simulink model "SIM_SAD_DEMO"  (R2025b)
settings: Solver=ode5  StartTime=0.0  StopTime=2*T  FixedStep=0.1  RelTol=1e-3
model workspace (MAT data in the model file):
  Pnull = Simulink.Parameter
  Pnull.Value = Simulink.data.Expression
  Pnull.Value.ExpressionString = "zeros(3,1)"
  Pnull.Complexity = 'real'
  Pnull.Dimensions = -1
  Pnull.DataType = 'auto'
  rho_albedo_medio = Simulink.Parameter
  rho_albedo_medio.Value = 0.3
  rho_albedo_medio.Complexity = 'real'
  rho_albedo_medio.Dimensions = [1 1]
  rho_albedo_medio.DataType = 'auto'
values from neighbouring files (symbols this model uses):
  Aree = zeros(10,1)    [SCRIPT_SAD_DEMO.m]
  base_seed = base_seed_MC + k    [SCRIPT_SAD_DEMO.m]
  c = astroConstants(5)*1e3    [SCRIPT_SAD_DEMO.m]
  draan = 1.99096871e-7    (= 1.99096871e-07)    [SCRIPT_SAD_DEMO.m]
  dwell_time = 30    [SCRIPT_SAD_DEMO.m]
  eps_att = deg2rad(0.2)    [SCRIPT_SAD_DEMO.m]
  eps_E = deg2rad(astroConstants(63))    [SCRIPT_SAD_DEMO.m]
  eps_h_r = 0.001    [SCRIPT_SAD_DEMO.m]
  eps_w = deg2rad(0.1)    [SCRIPT_SAD_DEMO.m]
  err_max = deg2rad(15)    [SCRIPT_SAD_DEMO.m]
  F_e = 1358    [SCRIPT_SAD_DEMO.m]
  h_r_max = 0.05    [SCRIPT_SAD_DEMO.m]
  h_r_safe = 0.001    [SCRIPT_SAD_DEMO.m]
  j_B = [0.01; 0.05; 0.01]    [SCRIPT_SAD_DEMO.m]
  J_depl = J_nom    [SCRIPT_SAD_DEMO.m]
  JD0 = juliandate(startTime)    [SCRIPT_SAD_DEMO.m]
  k_b = 200000    [SCRIPT_SAD_DEMO.m]
  Kd = K(:, 1:3)    [SCRIPT_SAD_DEMO.m]
  kep = [a,e,incl,raan,w,theta]    [SCRIPT_SAD_DEMO.m]
  Kp = K(:, 4:6)    [SCRIPT_SAD_DEMO.m]
  mu = astroConstants(13)    [SCRIPT_SAD_DEMO.m]
  n = sqrt( (mu/ (a)^3))    [SCRIPT_SAD_DEMO.m]
  n_sun = 2*pi/T_sun    (= 1.99238499086e-07)    [SCRIPT_SAD_DEMO.m]
  Nmat = [ ... (first row only)    [SCRIPT_SAD_DEMO.m]
  r_sun = 1*AU    [SCRIPT_SAD_DEMO.m]
  Re = astroConstants(23)    [SCRIPT_SAD_DEMO.m]
  rf = [ ... (first row only)    [SCRIPT_SAD_DEMO.m]
  rhod = 0.1*ones(10,1)    [SCRIPT_SAD_DEMO.m]
  rhos = zeros(10,1)    [SCRIPT_SAD_DEMO.m]
  SRP = SRP_nom    [SCRIPT_SAD_DEMO.m]
  theta = 0    [SCRIPT_SAD_DEMO.m]
  w0 = w0_nom    [SCRIPT_SAD_DEMO.m]
  w_enter = Control.w_tumbling    [SCRIPT_SAD_DEMO.m]
  w_enter_2 = Control.w_pointing    [SCRIPT_SAD_DEMO.m]
  w_exit = deg2rad(4)    [SCRIPT_SAD_DEMO.m]
  w_exit_2 = deg2rad(1.5)    [SCRIPT_SAD_DEMO.m]
undefined symbols (not defined in the file or in its folder): DiscIntNeverNeededParam, Filter, Gyro, Magmeter, MTQ, q, RW, Sun_sensor
libraries: matrix_library x41, LIBRARY_SAD x40, simulink x1, cstblocks x1
(part 1 of 4)
settings Model: Creator=fabio  LastModifiedBy=delil

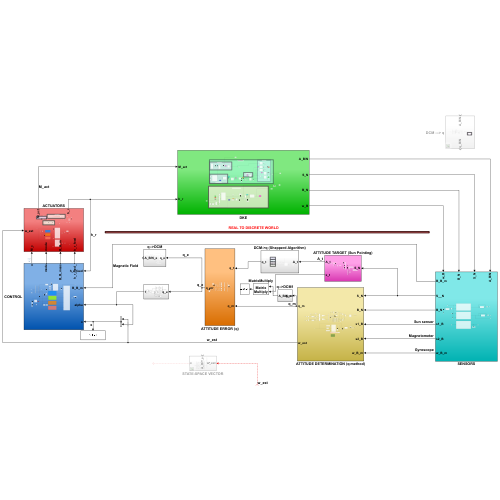
[thumbnail: Simulink's stored preview of the top-level diagram]
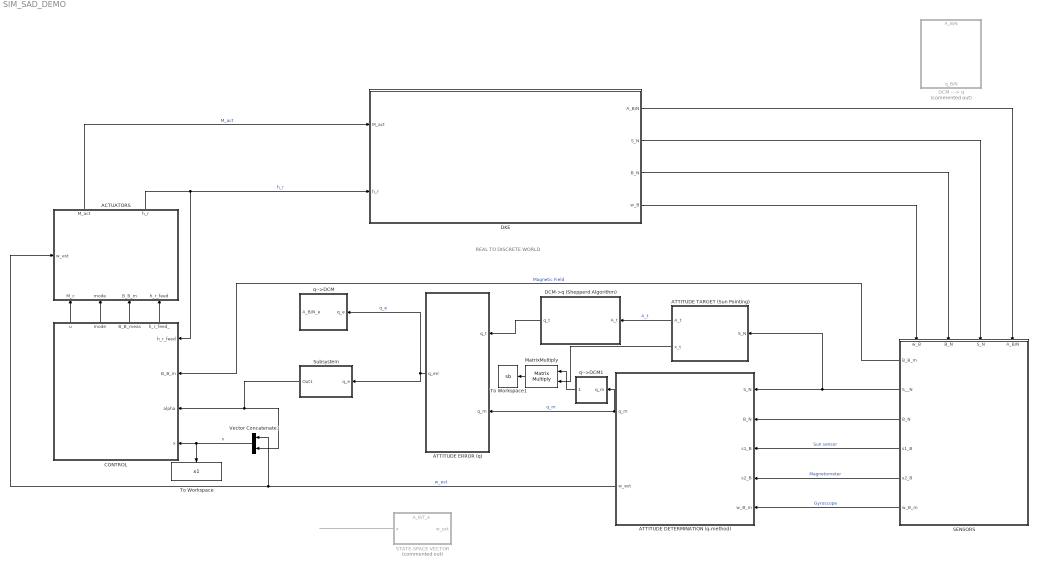
== system SIM_SAD_DEMO ==
  note: REAL TO DISCRETE WORLD
  ACTUATORS : Subsystem
      settings: PortSchema="{\"entries\":[{\"content\":{\"sides\":[{\"content\":{\"connectorIds\":[\"In1\",\"In2\",\"In3\",\"In4\"]},\"type\":\"ConnectorPlacement.EquallySpacedRectSide\",\"uuid\":\"6f22ed06-999b-49a4-bbcf-c00740f0bb3e\"},{\"content\":{\"connectorIds\":[\"Out1\",\"Out2\"],\"side\":\"RIGHT\"},\"type\":\"ConnectorPlacement.EquallySpacedRectSide\",\"uuid\":\"a2723920-c354-4b44-95a5-a047723a6fce\"},{\"content\":{\"connectorIds\":[\"In5\"],\"side\":\"TOP\"},\"type\":\"ConnectorPlacement.EquallySpacedRectSide\",\"uuid\":\"3a79ee58-4fdd-4e66-816d-19ecec84d660\"},{\"content\":{\"side\":\"BOTTOM\"},\"type\":\"ConnectorPlacement.EquallySpacedRectSide\",\"uuid\":\"88529345-5c62-4e9f-9741-99c35e09ad49\"}]},\"type\":\"ConnectorPlacement.EquallySpacedConnector\",\"uuid\":\"ec6e585e-60d6-43a1-884b-cd7dbc18dea8\"}],\"packageUris\":[\"http://schema.mathworks.com/mf0/Connector/R2020b\"],\"version\":\"1.0\"}"
  ATTITUDE DETERMINATION (q-method) : Subsystem
  ATTITUDE ERROR (q) : Subsystem
  ATTITUDE TARGET (Sun Pointing) : Subsystem
  CONTROL : Subsystem
      settings: PortSchema="{\"entries\":[{\"content\":{\"sides\":[{\"content\":{},\"type\":\"ConnectorPlacement.EquallySpacedRectSide\",\"uuid\":\"883b2e58-b302-40a6-9310-8bc36577f20a\"},{\"content\":{\"connectorIds\":[\"Out1\",\"Out2\",\"Out3\",\"Out4\"],\"side\":\"RIGHT\"},\"type\":\"ConnectorPlacement.EquallySpacedRectSide\",\"uuid\":\"3f5ac81e-dbcc-48df-b297-a852c6b84cd5\"},{\"content\":{\"side\":\"TOP\"},\"type\":\"ConnectorPlacement.EquallySpacedRectSide\",\"uuid\":\"b9661aa9-e9e6-4933-8b5a-68fb8ed8b613\"},{\"content\":{\"connectorIds\":[\"In1\",\"In2\",\"In3\",\"In4\"],\"side\":\"BOTTOM\"},\"type\":\"ConnectorPlacement.EquallySpacedRectSide\",\"uuid\":\"f58abdc6-33e7-496f-818d-03ad59e960e0\"}]},\"type\":\"ConnectorPlacement.EquallySpacedConnector\",\"uuid\":\"d8cd4486-f7c8-49c6-99e5-77f1928d07fe\"}],\"packageUris\":[\"http://schema.mathworks.com/mf0/Connector/R2020b\"],\"version\":\"1.0\"}"
  DCM ---> q : Subsystem  Commented=on
  DCM->q (Shepperd Algorithm) : Subsystem
  DKE : Subsystem
  MatrixMultiply : Product  Multiplication=Matrix(*)
  SENSORS : Subsystem
      settings: PortSchema="{\"entries\":[{\"content\":{\"sides\":[{\"content\":{\"connectorIds\":[\"In1\",\"In2\",\"In3\",\"In4\"]},\"type\":\"ConnectorPlacement.EquallySpacedRectSide\",\"uuid\":\"40962b30-3bcb-49e0-bc68-6aa3a31cfc97\"},{\"content\":{\"side\":\"RIGHT\"},\"type\":\"ConnectorPlacement.EquallySpacedRectSide\",\"uuid\":\"a8221d80-3d13-495d-884e-34f2ccc75f25\"},{\"content\":{\"connectorIds\":[\"Out1\",\"Out2\",\"Out3\",\"Out4\",\"Out5\",\"Out6\"],\"side\":\"TOP\"},\"type\":\"ConnectorPlacement.EquallySpacedRectSide\",\"uuid\":\"62b0f620-b15f-4d6a-bcfa-939a48d36217\"}]},\"type\":\"ConnectorPlacement.EquallySpacedConnector\",\"uuid\":\"bc93d320-282b-4258-8528-17688a47c52b\"}],\"packageUris\":[\"http://schema.mathworks.com/mf0/Connector/R2020b\"],\"version\":\"1.0\"}"
  STATE-SPACE VECTOR : Subsystem  Commented=on
      settings: PortSchema="{\"entries\":[{\"content\":{\"sides\":[{\"content\":{\"connectorIds\":[\"In1\"]},\"type\":\"ConnectorPlacement.EquallySpacedRectSide\",\"uuid\":\"179348e5-c488-47fb-b567-6c698cd263cb\"},{\"content\":{\"connectorIds\":[\"Out1\"],\"side\":\"RIGHT\"},\"type\":\"ConnectorPlacement.EquallySpacedRectSide\",\"uuid\":\"b2471475-7911-4c4c-b1de-354e85644b05\"},{\"content\":{\"connectorIds\":[\"In2\"],\"side\":\"TOP\"},\"type\":\"ConnectorPlacement.EquallySpacedRectSide\",\"uuid\":\"d61f0b2a-82cf-4d0f-843a-7dc5d306adfe\"},{\"content\":{\"side\":\"BOTTOM\"},\"type\":\"ConnectorPlacement.EquallySpacedRectSide\",\"uuid\":\"cf78bb57-5448-49c7-a009-bc1da3dda3c1\"}]},\"type\":\"ConnectorPlacement.EquallySpacedConnector\",\"uuid\":\"246de782-537f-47b1-b071-25d14f8cca05\"}],\"packageUris\":[\"http://schema.mathworks.com/mf0/Connector/R2020b\"],\"version\":\"1.0\"}"
  Subsystem : Subsystem
  To Workspace : ToWorkspace  VariableName=x1  SampleTime=-1
  To Workspace1 : ToWorkspace  VariableName=sb  SampleTime=-1
  Vector Concatenate1 : Concatenate
  q-->DCM : Subsystem
  q-->DCM1 : Subsystem
  wires:
  MatrixMultiply/1 -> To Workspace1/1
  SENSORS/1(B_B_m) -> CONTROL/3(B_B_m)  "Magnetic Field"
  Vector Concatenate1/1 -> To Workspace/1, CONTROL/1(x)  "x"
  DKE/1(A_B/N) -> SENSORS/4(A_B/N)
  DKE/2(S_N) -> SENSORS/3(S_N)
  SENSORS/3(B_N) -> ATTITUDE DETERMINATION (q-method)/2(B_N)
  CONTROL/2(mode) -> ACTUATORS/2(mode)
  ATTITUDE TARGET (Sun Pointing)/1(A_t) -> DCM->q (Shepperd Algorithm)/1(A_t)  "A_t"
  ATTITUDE DETERMINATION (q-method)/1(q_m) -> ATTITUDE ERROR (q)/2(q_m), q-->DCM1/1(q_m)  "q_m"
  CONTROL/4(h_r_feed_) -> ACTUATORS/4(h_r_feed)
  SENSORS/5(s2_B) -> ATTITUDE DETERMINATION (q-method)/4(s2_B)  "Magnetometer"
  DKE/4(w_B) -> SENSORS/1(w_B)
  SENSORS/2(S__N) -> ATTITUDE TARGET (Sun Pointing)/1(S_N), ATTITUDE DETERMINATION (q-method)/1(S_N)
  ATTITUDE ERROR (q)/1(q_err) -> q-->DCM/1(q_e), Subsystem/1(q_e)  "q_e"
  DCM->q (Shepperd Algorithm)/1(q_t) -> ATTITUDE ERROR (q)/1(q_t)
  Subsystem/1(Out1) -> Vector Concatenate1/2, CONTROL/2(alpha)
  CONTROL/1(u) -> ACTUATORS/1(M_c)
  ACTUATORS/1(M_act) -> DKE/1(M_act)  "M_act"
  CONTROL/3(B_B_meas) -> ACTUATORS/3(B_B_m)
  SENSORS/6(w_B_m) -> ATTITUDE DETERMINATION (q-method)/5(w_B_m)  "Gyroscope"
  ? -> STATE-SPACE VECTOR/1(w_est)  "w_est"
  ATTITUDE TARGET (Sun Pointing)/2(x_t) -> MatrixMultiply/2
  DKE/3(B_N) -> SENSORS/2("B_N ")
  ACTUATORS/2(h_r) -> DKE/2(h_r), CONTROL/4(h_r_feed)  "h_r"
  ATTITUDE DETERMINATION (q-method)/2(w_est) -> ACTUATORS/5(w_est), Vector Concatenate1/1  "w_est"
  STATE-SPACE VECTOR/1(x) -> ?
  SENSORS/4(s1_B) -> ATTITUDE DETERMINATION (q-method)/3(s1_B)  "Sun sensor"
  q-->DCM1/1(A_B/N_m) -> MatrixMultiply/1

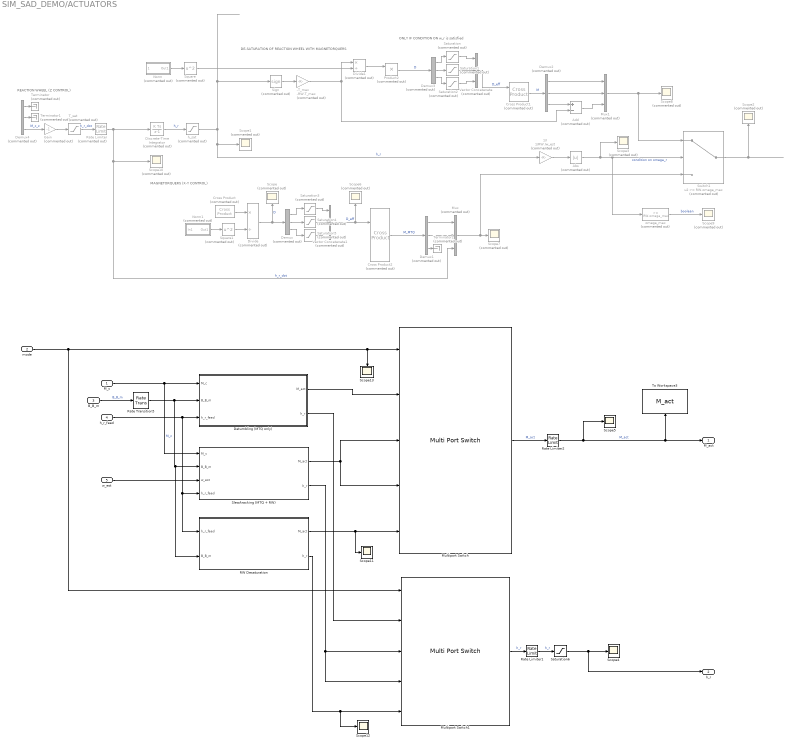
== system SIM_SAD_DEMO/ACTUATORS ==
  note: ONLY IF CONDITION ON w_r is satisfied
  note: DE-SATURATION OF REACTION WHEEL WITH MAGNETORQUERS
  note: REACTION WHEEL (Z CONTROL)
  note: MAGNETORQUERS (X-Y CONTROL)
  M_c : Inport
  mode : Inport  Port=2
  B_B_m : Inport  Port=3
  h_r_feed : Inport  Port=4
  w_est : Inport  Port=5
  -T_max : Gain  Commented=on  Gain=-RW.T_max
  1/I : Gain  Commented=on  Gain=1/RW.Iw_est
  Abs : Abs  Commented=on  SaturateOnIntegerOverflow=off
  Add : Sum  Commented=on  Inputs=+-
  Cross Product : matrix_library/Cross Product  Commented=on
  Cross Product1 : matrix_library/Cross Product  Commented=on
  Cross Product2 : matrix_library/Cross Product  Commented=on
  Demux{,1..4} (5 alike) : Demux  Commented=on  Outputs=3
  Detumbling (MTQ only) : Subsystem
  Discrete-Time Integrator : DiscreteIntegrator  Commented=on  SampleTime=-1  ICPrevOutput=DiscIntNeverNeededParam  ICPrevScaledInput=DiscIntNeverNeededParam
  Divide : Product  Commented=on  Inputs=*/
  Divide1 : Product  Commented=on  Inputs=*/
  Gain : Gain  Commented=on  Gain=-1
  Multiport Switch : MultiPortSwitch  Inputs=4  DiagnosticForDefault=None  SaturateOnIntegerOverflow=off  InputSameDT=off
  Multiport Switch1 : MultiPortSwitch  Inputs=4  DiagnosticForDefault=None  SaturateOnIntegerOverflow=off  InputSameDT=off
  Mux : Mux  Commented=on  Inputs=3
  Mux1 : Mux  Commented=on  Inputs=3
  Norm : Subsystem  Commented=on
  Norm1 : Subsystem  Commented=on
  Product2 : Product  Commented=on
  RW Desaturation : Subsystem
  Rate Limiter : RateLimiter  Commented=on  RisingSlewLimit=200  FallingSlewLimit=-200  SampleTimeMode=inherited
  Rate Limiter1 : RateLimiter  SampleTimeMode=inherited
  Rate Limiter2 : RateLimiter  SampleTimeMode=inherited
  Rate Transition5 : RateTransition  OutPortSampleTime=max([Sun_sensor.Ts,Magmeter.Ts,Gyro.Ts])
  Saturation{,1,3..4} (4 alike) : Saturate  Commented=on  UpperLimit=MTQ.D_max_XY  LowerLimit=-MTQ.D_max_XY
  Saturation2 : Saturate  Commented=on  UpperLimit=MTQ.D_max_Z  LowerLimit=-MTQ.D_max_Z
  Saturation5 : Saturate  Commented=on  UpperLimit=MTQ.D_max_Z  LowerLimit=-MTQ.D_max_Z
  Saturation6 : Saturate  UpperLimit=RW.h_max  LowerLimit=-RW.h_max
  Scope{,1..3,6..10} (9 alike) : Scope  Commented=on
      Scope settings: ActiveDisplayYMinimum=-14.411553950631344  ActiveDisplayYMaximum=16.201380468990443  DataLoggingVariableName=ScopeData98
      Scope1 settings: ActiveDisplayYMinimum=-0.0062499999999999986  ActiveDisplayYMaximum=0.05625  DataLoggingVariableName=ScopeData104
      Scope10 settings: ActiveDisplayYMinimum=-0.0099459564386370769  ActiveDisplayYMaximum=0.0095136079477336766  DataLoggingVariableName=ScopeData110
      Scope2 settings: ActiveDisplayYMinimum=-9.87718527241468E-5  ActiveDisplayYMaximum=8.9550339314577583E-5  DataLoggingVariableName=ScopeData102
      Scope3 settings: ActiveDisplayYMinimum=-65.022890693082175  ActiveDisplayYMaximum=585.20601623773973  DataLoggingVariableName=ScopeData60
      Scope6 settings: ActiveDisplayYMinimum=-0.625  ActiveDisplayYMaximum=0.625  DataLoggingVariableName=ScopeData101
      Scope7 settings: ActiveDisplayYMinimum=-1  ActiveDisplayYMaximum=1  DataLoggingVariableName=ScopeData100
      Scope8 settings: ActiveDisplayYMinimum=-0.001101814270019531  ActiveDisplayYMaximum=0.00911127471923828  DataLoggingVariableName=ScopeData103
      Scope9 settings: ActiveDisplayYMinimum=-0.12499999999999997  ActiveDisplayYMaximum=1.125  DataLoggingVariableName=ScopeData107
  Scope{4..5,11..13} (5 alike) : Scope
      Scope11 settings: ActiveDisplayYMinimum=-1  ActiveDisplayYMaximum=1  DataLoggingVariableName=ScopeData119
      Scope12 settings: ActiveDisplayYMinimum=-1  ActiveDisplayYMaximum=1  DataLoggingVariableName=ScopeData121
      Scope13 settings: ActiveDisplayYMinimum=-0.49999999999999989  ActiveDisplayYMaximum=4.5  DataLoggingVariableName=ScopeData125
      Scope4 settings: ActiveDisplayYMinimum=-0.0625  ActiveDisplayYMaximum=0.0625  DataLoggingVariableName=ScopeData114
      Scope5 settings: ActiveDisplayYMinimum=-1.2499999497669214  ActiveDisplayYMaximum=1.2499999579450596  DataLoggingVariableName=ScopeData115
  Sign : Signum  Commented=on
  Slew/tracking (MTQ + RW) : Subsystem
  Square : Math  Commented=on  Operator=square
  Square1 : Math  Commented=on  Operator=square
  Switch1 : Switch  Commented=on  Threshold=RW.omega_max  SaturateOnIntegerOverflow=off  InputSameDT=off
  T_sat : Saturate  Commented=on  UpperLimit=RW.T_max  LowerLimit=-RW.T_max
  Terminator : Terminator  Commented=on
  Terminator1 : Terminator  Commented=on
  Terminator2 : Terminator  Commented=on
  To Workspace3 : ToWorkspace  VariableName=M_act  SampleTime=-1
  Vector Concatenate : Concatenate  Commented=on  NumInputs=3
  Vector Concatenate1 : Concatenate  Commented=on  NumInputs=3
  h_sat : Saturate  Commented=on  UpperLimit=RW.h_max  LowerLimit=-RW.h_max
  omega_max : simulink/Logic and Bit Operations/Compare To Constant  Commented=on  relop=>=  const=RW.omega_max  OutDataTypeStr=boolean
  M_act : Outport
  h_r : Outport  Port=2
  wires:
  Discrete-Time Integrator/1 -> h_sat/1  "h_r"
  Demux3/1 -> Saturation/1
  Demux3/3 -> Saturation2/1
  Product2/1 -> Demux3/1  "D"
  Divide1/1 -> Product2/1
  -T_max/1 -> Add/2, Divide1/1
  Mux1/1 -> Scope8/1, Switch1/1
  Norm/1(Out1) -> Square/1
  Saturation2/1 -> Vector Concatenate/3
  Saturation/1 -> Vector Concatenate/1
  Cross Product1/1 -> Demux2/1  "M"
  Vector Concatenate/1 -> Cross Product1/1  "D_eff"
  Demux3/2 -> Saturation1/1
  Add/1 -> Mux1/3
  Sign/1 -> -T_max/1
  T_sat/1 -> Rate Limiter/1  "h_r_dot"
  ? -> Norm1/1(In1), Cross Product/1, Cross Product2/2, Cross Product1/2, Product2/2, Norm/1(B_B_m)  "B_B_m"
  Demux4/3 -> Gain/1  "M_c_z"
  Demux2/3 -> Add/1
  Demux2/2 -> Mux1/2
  Demux2/1 -> Mux1/1
  1/I/1 -> Abs/1
  Abs/1 -> omega_max/1, Switch1/2, Scope3/1  "condition on omega_r"
  Saturation1/1 -> Vector Concatenate/2
  Cross Product/1 -> Divide/1
  Demux/1 -> Saturation3/1
  Vector Concatenate1/1 -> Cross Product2/1, Scope6/1  "D_eff"
  Saturation4/1 -> Vector Concatenate1/2
  Square1/1 -> Divide/2
  Norm1/1(Out1) -> Square1/1
  ? -> Demux4/1, Cross Product/2  "M_c"
  Divide/1 -> Scope/1, Demux/1  "D"
  Demux/2 -> Saturation4/1
  Saturation3/1 -> Vector Concatenate1/1
  Demux/3 -> Saturation5/1
  omega_max/1 -> Scope9/1  "boolean"
  Square/1 -> Divide1/2
  Saturation5/1 -> Vector Concatenate1/3
  Cross Product2/1 -> Demux1/1  "M_MTQ"
  Demux1/1 -> Mux/1
  Demux1/2 -> Mux/2
  Mux/1 -> Scope7/1, Switch1/3
  Demux4/1 -> Terminator/1
  Demux4/2 -> Terminator1/1
  Demux1/3 -> Terminator2/1
  Switch1/1 -> Scope2/1
  h_sat/1 -> Sign/1, Scope1/1, 1/I/1  "h_r"
  Rate Limiter/1 -> Discrete-Time Integrator/1, Mux/3, Scope10/1  "h_r_dot"
  Gain/1 -> T_sat/1
  M_c/1 -> Slew/tracking (MTQ + RW)/1(M_c), Detumbling (MTQ only)/1(M_c)  "M_c"
  B_B_m/1 -> Rate Transition5/1  "B_B_m"
  h_r_feed/1 -> RW Desaturation/1(h_r_feed), Slew/tracking (MTQ + RW)/4(h_r_feed), Detumbling (MTQ only)/3(h_r_feed)
  Detumbling (MTQ only)/1(M_act) -> Multiport Switch/2
  Detumbling (MTQ only)/2(h_r) -> Multiport Switch1/2
  Multiport Switch/1 -> Rate Limiter2/1  "M_act"
  Multiport Switch1/1 -> Rate Limiter1/1  "h_r"
  w_est/1 -> Slew/tracking (MTQ + RW)/3(w_est)
  Slew/tracking (MTQ + RW)/1(M_act) -> Multiport Switch/4, Multiport Switch/3
  Slew/tracking (MTQ + RW)/2(h_r) -> Multiport Switch1/3, Multiport Switch1/4
  Rate Limiter1/1 -> Saturation6/1  "h_r"
  Rate Limiter2/1 -> Scope5/1, M_act/1, To Workspace3/1  "M_act"
  Saturation6/1 -> h_r/1, Scope4/1
  mode/1 -> Multiport Switch1/1, Multiport Switch/1, Scope13/1
  RW Desaturation/1(M_act) -> Multiport Switch/5, Scope11/1
  RW Desaturation/2(h_r) -> Multiport Switch1/5, Scope12/1
  Rate Transition5/1 -> RW Desaturation/2(B_B_m), Slew/tracking (MTQ + RW)/2(B_B_m), Detumbling (MTQ only)/2(B_B_m)

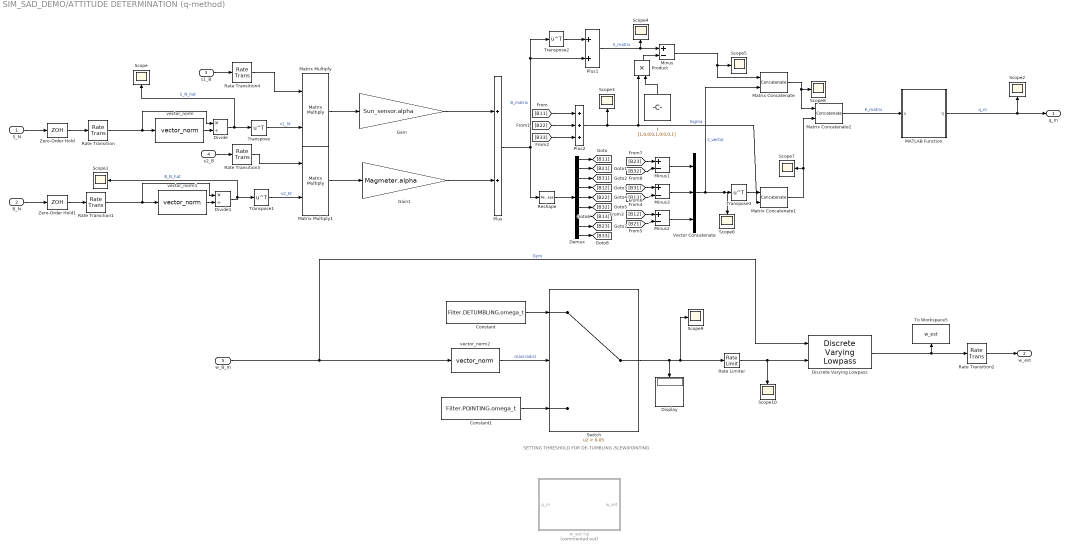
== system SIM_SAD_DEMO/ATTITUDE DETERMINATION (q-method) ==
  note: SETTING THRESHOLD FOR DE-TUMBLING /SLEW/POINTING
  S_N : Inport
  B_N : Inport  Port=2
  s1_B : Inport  Port=3
  s2_B : Inport  Port=4
  w_B_m : Inport  Port=5
  Constant : Constant  Value=Filter.DETUMBLING.omega_t
  Constant1 : Constant  Value=Filter.POINTING.omega_t
  Demux : Demux  Outputs=9
  Discrete Varying Lowpass : cstblocks/Linear Parameter Varying/Discrete Varying Lowpass  N=1  w0=0  Ts=Gyro.Ts
  Display : Display
  Divide : Product  Inputs=*/
  Divide1 : Product  Inputs=*/
  Gain : Gain  Gain=Sun_sensor.alpha
  Gain1 : Gain  Gain=Magmeter.alpha
  I : Constant  Value=[1,0,0;0,1,0;0,0,1]
  MATLAB Function : MATLAB Function  TreatAsAtomicUnit=on  SystemSampleTime=q.Ts
  Matrix Concatenate : Concatenate  Mode=Multidimensional array  ConcatenateDimension=2
  Matrix Concatenate1 : Concatenate  Mode=Multidimensional array  ConcatenateDimension=2
  Matrix Concatenate2 : Concatenate  Mode=Multidimensional array
  Matrix Multiply : Product  Multiplication=Matrix(*)
  Matrix Multiply1 : Product  Multiplication=Matrix(*)
  Minus{,1..3} (4 alike) : Sum  Inputs=+-
  Plus : Sum
  Plus1 : Sum
  Plus2 : Sum  Inputs=+++
  Product : Product
  Rate Limiter : RateLimiter  RisingSlewLimit=5  FallingSlewLimit=-5  SampleTimeMode=inherited  InitialCondition=Filter.DETUMBLING.omega_t
  Rate Transition{,1..4} (5 alike) : RateTransition  OutPortSampleTime=max([Sun_sensor.Ts,Magmeter.Ts,Gyro.Ts])
  Reshape : Reshape  OutputDimensionality=Customize  OutputDimensions=[9,1]
  Scope{,1..10} (11 alike) : Scope
      Scope settings: ActiveDisplayYMinimum=-0.12499999999999997  ActiveDisplayYMaximum=1.125  DataLoggingVariableName=ScopeData61
      Scope1 settings: ActiveDisplayYMinimum=-0.60786913937993192  ActiveDisplayYMaximum=1.0990417923572595  DataLoggingVariableName=ScopeData62
      Scope10 settings: ActiveDisplayYMinimum=0.40419161676646631  ActiveDisplayYMaximum=9.3562874251497  DataLoggingVariableName=ScopeData58
      Scope2 settings: ActiveDisplayYMinimum=-0.9533532616313245  ActiveDisplayYMaximum=1.1062124291352333  DataLoggingVariableName=ScopeData74
      Scope3 settings: ActiveDisplayYMinimum=-1  ActiveDisplayYMaximum=1  DataLoggingVariableName=ScopeData75
      Scope4 settings: DataLoggingVariableName=ScopeData76
      Scope5 settings: ActiveDisplayYMinimum=-1  ActiveDisplayYMaximum=1  DataLoggingVariableName=ScopeData77
      Scope6 settings: DataLoggingVariableName=ScopeData78
      Scope7 settings: ActiveDisplayYMinimum=-1  ActiveDisplayYMaximum=1  DataLoggingVariableName=ScopeData79
      Scope8 settings: ActiveDisplayYMinimum=-1.2343387282561236  ActiveDisplayYMaximum=1.1812725103052406  DataLoggingVariableName=ScopeData80
      Scope9 settings: ActiveDisplayYMinimum=-0.12499999999999978  ActiveDisplayYMaximum=11.125  DataLoggingVariableName=ScopeData85
  Switch : Switch  Criteria=u2 > Threshold  Threshold=0.05  SaturateOnIntegerOverflow=off  InputSameDT=off
  To Workspace5 : ToWorkspace  VariableName=w_est  SampleTime=-1
  Transpose{,1..3} (4 alike) : Math  Operator=transpose
  Vector Concatenate : Concatenate  NumInputs=3
  Zero-Order Hold : ZeroOrderHold  SampleTime=max([Sun_sensor.Ts,Magmeter.Ts,Gyro.Ts])
  Zero-Order Hold1 : ZeroOrderHold  SampleTime=max([Sun_sensor.Ts,Magmeter.Ts,Gyro.Ts])
  vector_norm : LIBRARY_SAD/vector_norm  SystemSampleTime=-1  VariantActivationTime=update diagram  EmptyChoice=off  PassThrough=off  PassThroughVariantControl=(default)  EmptyChoiceVariantControl=(default)  AllowFlexibleInterface=on  Latency=0  AutoFrameSizeCalculation=off
  vector_norm1 : LIBRARY_SAD/vector_norm  SystemSampleTime=-1  VariantActivationTime=update diagram  EmptyChoice=off  PassThrough=off  PassThroughVariantControl=(default)  EmptyChoiceVariantControl=(default)  AllowFlexibleInterface=on  Latency=0  AutoFrameSizeCalculation=off
  vector_norm2 : LIBRARY_SAD/vector_norm  SystemSampleTime=-1  VariantActivationTime=update diagram  EmptyChoice=off  PassThrough=off  PassThroughVariantControl=(default)  EmptyChoiceVariantControl=(default)  AllowFlexibleInterface=on  Latency=0  AutoFrameSizeCalculation=off
  w_est (q) : Subsystem  Commented=on
  q_m : Outport
  w_est : Outport  Port=2
  wires:
  vector_norm/1 -> Divide/2
  Demux/6 -> [B32]
  Divide/1 -> Scope/1, Transpose/1  "S_N_hat"
  Gain/1 -> Plus/1
  [B32] -> Minus1/2
  Gain1/1 -> Plus/2
  S_N/1 -> Zero-Order Hold/1
  Plus2/1 -> Scope3/1, Product/1, Matrix Concatenate1/2  "Sigma"
  B_N/1 -> Zero-Order Hold1/1
  Demux/4 -> [B12]
  Plus/1 -> Reshape/1, Transpose2/1, Plus1/2  "B_matrix"
  Divide1/1 -> Scope1/1, Transpose1/1  "B_N_hat"
  [B12] -> Minus2/1
  Demux/3 -> [B31]
  Demux/8 -> [B23]
  Vector Concatenate/1 -> Matrix Concatenate/2, Transpose3/1, Scope6/1  "z_vector"
  Minus1/1 -> Vector Concatenate/1
  Minus2/1 -> Vector Concatenate/3
  Transpose2/1 -> Plus1/1
  [B11] -> Plus2/1
  Transpose/1 -> Matrix Multiply/2  "v1_N'"
  Minus/1 -> Scope5/1, Matrix Concatenate/1
  Matrix Concatenate1/1 -> Scope7/1, Matrix Concatenate2/2
  Demux/1 -> [B11]
  [B22] -> Plus2/2
  Matrix Multiply1/1 -> Gain1/1
  Demux/2 -> [B21]
  [B23] -> Minus1/1
  Demux/5 -> [B22]
  Matrix Multiply/1 -> Gain/1
  Demux/9 -> [B33]
  Reshape/1 -> Demux/1
  Demux/7 -> [B13]
  vector_norm1/1 -> Divide1/2
  [B33] -> Plus2/3
  Matrix Concatenate/1 -> Matrix Concatenate2/1, Scope8/1
  Transpose1/1 -> Matrix Multiply1/2  "v2_N'"
  Transpose3/1 -> Matrix Concatenate1/1
  Minus3/1 -> Vector Concatenate/2
  [B31] -> Minus3/1
  Plus1/1 -> Minus/1, Scope4/1  "S_matrix"
  [B13] -> Minus3/2
  [B21] -> Minus2/2
  Product/1 -> Minus/2
  I/1 -> Product/2
  s1_B/1 -> Rate Transition4/1
  s2_B/1 -> Rate Transition3/1
  MATLAB Function/1(q) -> q_m/1, Scope2/1  "q_m"
  Switch/1 -> Rate Limiter/1, Scope9/1, Display/1
  Matrix Concatenate2/1 -> MATLAB Function/1(u)  "K_matrix"
  vector_norm2/1 -> Switch/2  "max(rad/s)"
  w_B_m/1 -> vector_norm2/1, Discrete Varying Lowpass/1  "Gyro"
  Discrete Varying Lowpass/1 -> To Workspace5/1, Rate Transition2/1
  Constant/1 -> Switch/1
  Constant1/1 -> Switch/3
  Rate Limiter/1 -> Scope10/1, Discrete Varying Lowpass/2
  Rate Transition/1 -> Divide/1, vector_norm/1
  Rate Transition1/1 -> Divide1/1, vector_norm1/1
  Rate Transition3/1 -> Matrix Multiply1/1
  Rate Transition4/1 -> Matrix Multiply/1
  Zero-Order Hold/1 -> Rate Transition/1
  Zero-Order Hold1/1 -> Rate Transition1/1
  Rate Transition2/1 -> w_est/1

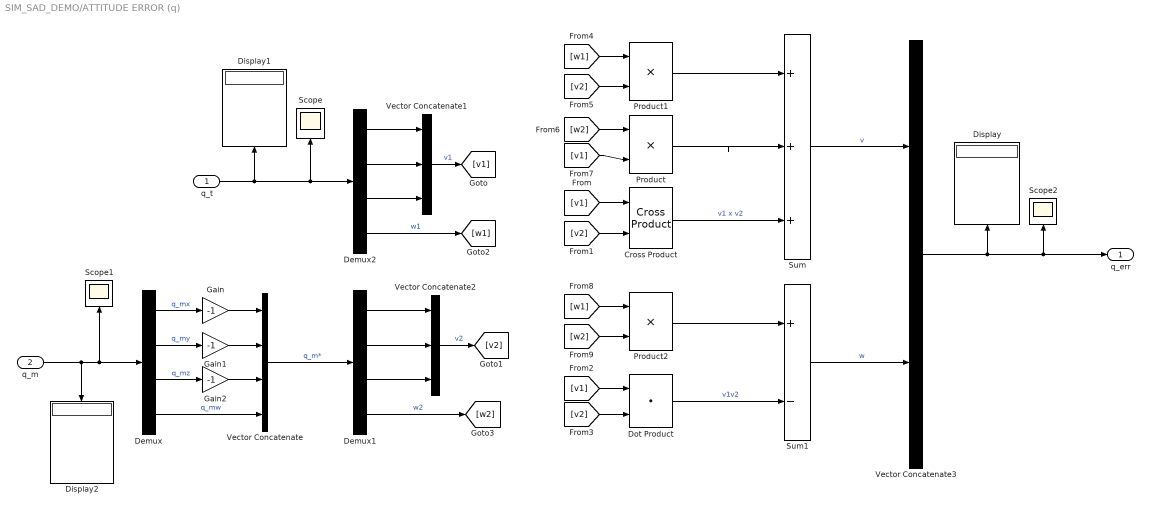
== system SIM_SAD_DEMO/ATTITUDE ERROR (q) ==
  q_t : Inport
  q_m : Inport  Port=2
  Cross Product : matrix_library/Cross Product
  Demux : Demux
  Demux1 : Demux
  Demux2 : Demux
  Display : Display
  Display1 : Display
  Display2 : Display
  Dot Product : DotProduct  OutDataTypeStr=Inherit: Inherit via internal rule
  Gain : Gain  Gain=-1
  Gain1 : Gain  Gain=-1
  Gain2 : Gain  Gain=-1
  Product : Product
  Product1 : Product
  Product2 : Product
  Scope : Scope
      settings: ActiveDisplayYMinimum=-0.12923710595911297  ActiveDisplayYMaximum=1.1085905151201327  DataLoggingVariableName=ScopeData63
  Scope1 : Scope
      settings: ActiveDisplayYMinimum=-1.1944830769885011  ActiveDisplayYMaximum=1.2235445279118087  DataLoggingVariableName=ScopeData64
  Scope2 : Scope
      settings: ActiveDisplayYMinimum=-1  ActiveDisplayYMaximum=1  DataLoggingVariableName=ScopeData65
  Sum : Sum  Inputs=+++
  Sum1 : Sum  Inputs=+-
  Vector Concatenate : Concatenate  NumInputs=4
  Vector Concatenate1 : Concatenate  NumInputs=3
  Vector Concatenate2 : Concatenate  NumInputs=3
  Vector Concatenate3 : Concatenate
  q_err : Outport
  wires:
  q_m/1 -> Scope1/1, Demux/1, Display2/1
  q_t/1 -> Demux2/1, Scope/1, Display1/1
  Demux/1 -> Gain/1  "q_mx"
  Demux/2 -> Gain1/1  "q_my"
  Demux/3 -> Gain2/1  "q_mz"
  Demux/4 -> Vector Concatenate/4  "q_mw"
  Gain2/1 -> Vector Concatenate/3
  Gain1/1 -> Vector Concatenate/2
  Gain/1 -> Vector Concatenate/1
  Vector Concatenate/1 -> Demux1/1  "q_m*"
  Demux1/1 -> Vector Concatenate2/1
  Demux1/2 -> Vector Concatenate2/2
  Demux1/3 -> Vector Concatenate2/3
  Demux1/4 -> [w2]  "w2"
  Demux2/1 -> Vector Concatenate1/1
  Demux2/2 -> Vector Concatenate1/2
  Demux2/3 -> Vector Concatenate1/3
  Vector Concatenate1/1 -> [v1]  "v1"
  Demux2/4 -> [w1]  "w1"
  Cross Product/1 -> Sum/3  "v1 x v2"
  Dot Product/1 -> Sum1/2  "v1v2"
  [v1] -> Cross Product/1
  Vector Concatenate2/1 -> [v2]  "v2"
  [v2] -> Cross Product/2
  [v1] -> Dot Product/1
  [v2] -> Dot Product/2
  [w1] -> Product1/1
  [v2] -> Product1/2
  [v1] -> Product/2
  [w2] -> Product/1
  Product1/1 -> Sum/1
  Product/1 -> Sum/2
  [w1] -> Product2/1
  [w2] -> Product2/2
  Product2/1 -> Sum1/1
  Sum/1 -> Vector Concatenate3/1  "v"
  Sum1/1 -> Vector Concatenate3/2  "w"
  Vector Concatenate3/1 -> q_err/1, Scope2/1, Display/1

== system SIM_SAD_DEMO/ATTITUDE TARGET (Sun Pointing) ==
  note: BORESIGHT AXIS : axis which points the Sun
  S_N : Inport
  Constant{1..2,4,6,8..11} (8 alike) : Constant  Value=0
  Constant{3,5,7,12} (4 alike) : Constant
  Cross Product : matrix_library/Cross Product
  Cross Product1 : matrix_library/Cross Product
  Display : Display
  Display1 : Display
  MatrixMultiply : Product  Multiplication=Matrix(*)
  Normalized Vector : Subsystem
  Normalized Vector2 : Subsystem
  Rate Transition3 : RateTransition  OutPortSampleTime=max([Sun_sensor.Ts,Magmeter.Ts,Gyro.Ts])
  Scope{,1..4} (5 alike) : Scope
      Scope settings: ActiveDisplayYMinimum=-0.12499999999999997  ActiveDisplayYMaximum=1.125  DataLoggingVariableName=ScopeData62
      Scope1 settings: ActiveDisplayYMinimum=-1  ActiveDisplayYMaximum=1  DataLoggingVariableName=ScopeData66
      Scope2 settings: ActiveDisplayYMinimum=-1  ActiveDisplayYMaximum=1  DataLoggingVariableName=ScopeData69
      Scope3 settings: ActiveDisplayYMinimum=-1  ActiveDisplayYMaximum=1  DataLoggingVariableName=ScopeData70
      Scope4 settings: ActiveDisplayYMinimum=-1  ActiveDisplayYMaximum=1  DataLoggingVariableName=ScopeData73
  Sum : Sum  Inputs=|+-
  Transpose : Math  Operator=transpose
  Vector Concatenate : Concatenate  NumInputs=3  Mode=Multidimensional array  ConcatenateDimension=2
  Vector Concatenate{1..4} (4 alike) : Concatenate  NumInputs=3
  Vector Concatenate5 : Concatenate  NumInputs=3  Mode=Multidimensional array  ConcatenateDimension=2
  Zero-Order Hold2 : ZeroOrderHold  SampleTime=max([Sun_sensor.Ts,Magmeter.Ts,Gyro.Ts])
  A_t : Outport
  x_t : Outport  Port=2
  wires:
  S_N/1 -> Zero-Order Hold2/1
  Normalized Vector2/1(s2_B) -> x_t/1, Cross Product/2, Cross Product1/1, Vector Concatenate/1, Scope/1  "x_t_hat"
  Vector Concatenate1/1 -> Cross Product/1  "k_hat"
  Cross Product/1 -> Normalized Vector/1(In1)
  Normalized Vector/1(Out1) -> Scope1/1, Vector Concatenate/2, Cross Product1/2  "y_t_hat"
  Cross Product1/1 -> Scope2/1, Vector Concatenate/3  "z_t_hat"
  Transpose/1 -> MatrixMultiply/1
  MatrixMultiply/1 -> Sum/1
  Vector Concatenate5/1 -> Display1/1, Sum/2  "I_matrix"
  Sum/1 -> Scope3/1
  Constant2/1 -> Vector Concatenate1/2
  Constant1/1 -> Vector Concatenate1/1
  Constant3/1 -> Vector Concatenate1/3
  Constant6/1 -> Vector Concatenate2/3
  Constant4/1 -> Vector Concatenate2/1
  Constant5/1 -> Vector Concatenate2/2
  Constant8/1 -> Vector Concatenate3/2
  Constant7/1 -> Vector Concatenate3/1
  Constant9/1 -> Vector Concatenate3/3
  Constant11/1 -> Vector Concatenate4/2
  Constant10/1 -> Vector Concatenate4/1
  Constant12/1 -> Vector Concatenate4/3
  Vector Concatenate3/1 -> Vector Concatenate5/1
  Vector Concatenate2/1 -> Vector Concatenate5/2
  Vector Concatenate4/1 -> Vector Concatenate5/3
  Vector Concatenate/1 -> A_t/1, Scope4/1, MatrixMultiply/2, Transpose/1, Display/1  "A_T_N"
  Zero-Order Hold2/1 -> Rate Transition3/1
  Rate Transition3/1 -> Normalized Vector2/1(r)

== system SIM_SAD_DEMO/CONTROL ==
  x : Inport
  alpha : Inport  Port=2
  B_B_m : Inport  Port=3
  h_r_feed : Inport  Port=4
  B_dot (Detumbling) : Subsystem
  Chart : Stateflow chart  TreatAsAtomicUnit=on  SystemSampleTime=q.Ts
  Delay : Delay  DelayLength=1  SampleTime=q.Ts
  Demux : Demux  Outputs=6
  ERROR VECTOR : Subsystem  Commented=on
  Multiport Switch : MultiPortSwitch  Inputs=4  DiagnosticForDefault=None  SaturateOnIntegerOverflow=off  InputSameDT=off
  RW Desaturation : Subsystem
  Rate Limiter : RateLimiter  RisingSlewLimit=5  FallingSlewLimit=-5  SampleTimeMode=inherited
  Rate Transition5 : RateTransition  OutPortSampleTime=max([Sun_sensor.Ts,Magmeter.Ts,Gyro.Ts])
  Scope : Scope  Commented=on
      settings: ActiveDisplayYMinimum=-0.12498972582518562  ActiveDisplayYMaximum=1.1249988581209451  DataLoggingVariableName=ScopeData105
  Scope1 : Scope
      settings: ActiveDisplayYMinimum=-0.49999999999999989  ActiveDisplayYMaximum=4.5  DataLoggingVariableName=ScopeData95
  Scope2 : Scope
      settings: ActiveDisplayYMinimum=-0.064681206847813172  ActiveDisplayYMaximum=0.60551119291621791  DataLoggingVariableName=ScopeData106
  Scope3 : Scope
      settings: ActiveDisplayYMinimum=-1.482622282484364  ActiveDisplayYMaximum=1.4697315712163508  DataLoggingVariableName=ScopeData55
  Slew Manouvre/pointing : Subsystem
  To Workspace1 : ToWorkspace  VariableName=u  SampleTime=-1
  Tracking : Subsystem
  Vector Concatenate : Concatenate  NumInputs=3
  Vector Concatenate1 : Concatenate  NumInputs=3
  vector_norm1 : LIBRARY_SAD/vector_norm  SystemSampleTime=-1  VariantActivationTime=update diagram  EmptyChoice=off  PassThrough=off  PassThroughVariantControl=(default)  EmptyChoiceVariantControl=(default)  AllowFlexibleInterface=on  Latency=0  AutoFrameSizeCalculation=off
  vector_norm2 : LIBRARY_SAD/vector_norm  SystemSampleTime=-1  VariantActivationTime=update diagram  EmptyChoice=off  PassThrough=off  PassThroughVariantControl=(default)  EmptyChoiceVariantControl=(default)  AllowFlexibleInterface=on  Latency=0  AutoFrameSizeCalculation=off
  vector_norm3 : LIBRARY_SAD/vector_norm  SystemSampleTime=-1  VariantActivationTime=update diagram  EmptyChoice=off  PassThrough=off  PassThroughVariantControl=(default)  EmptyChoiceVariantControl=(default)  AllowFlexibleInterface=on  Latency=0  AutoFrameSizeCalculation=off
  u : Outport
  mode : Outport  Port=2
  B_B_meas : Outport  Port=3
  h_r_feed_ : Outport  Port=4
  wires:
  x/1 -> Scope3/1, Demux/1
  Demux/1 -> Vector Concatenate/1  "w_x"
  Demux/2 -> Vector Concatenate/2  "w_y"
  Demux/3 -> Vector Concatenate/3  "w_z"
  Vector Concatenate/1 -> vector_norm3/1, Tracking/1(w_est), Slew Manouvre/pointing/1(w_est), B_dot (Detumbling)/1(w_est)  "w_est"
  B_dot (Detumbling)/1(M_c_detumbling) -> Multiport Switch/2  "DETUMBLING"
  B_B_m/1 -> Rate Transition5/1, B_B_meas/1
  Multiport Switch/1 -> Rate Limiter/1
  Slew Manouvre/pointing/1(Mc_slew) -> Multiport Switch/3  "SLEW"
  Tracking/1(Mc_tracking) -> Multiport Switch/4  "TRACKING"
  Rate Limiter/1 -> u/1, To Workspace1/1
  ERROR VECTOR/1(as) -> ?
  Demux/4 -> Vector Concatenate1/1  "alpha_x"
  Demux/5 -> Vector Concatenate1/2  "alpha_y"
  Demux/6 -> Vector Concatenate1/3  "alpha_z"
  alpha/1 -> vector_norm2/1, Slew Manouvre/pointing/2(as), ERROR VECTOR/1(A_B/T_e)
  Vector Concatenate1/1 -> vector_norm1/1, Tracking/2(alpha)  "alpha"
  Chart/1(mode) -> Multiport Switch/1, mode/1, Scope1/1  "mode"
  vector_norm1/1 -> [err_att_track]
  ? -> Scope/1
  vector_norm3/1 -> Chart/1(norm_w), Scope2/1
  [err_att_slew] -> Chart/2(err_att_slew)
  [err_att_track] -> Chart/3(err_att_track)
  RW Desaturation/1(M_c_desat) -> Multiport Switch/5  "DESATURATION"
  Delay/1 -> Chart/4(h_r_feed)
  Rate Transition5/1 -> B_dot (Detumbling)/2(B_B_m)
  h_r_feed/1 -> Delay/1, h_r_feed_/1
  vector_norm2/1 -> [err_att_slew]

== system SIM_SAD_DEMO/DCM ---> q ==
  note: CHECK BY RECONSTRUCTING A_B/N AND ORTHONORMALITY ERROR
  A_B/N : Inport
  Constant : Constant
  Demux : Demux  Outputs=9
  Divide{,1..3} (4 alike) : Product  Inputs=*/
  Gain : Gain  Gain=4
  Gain1 : Gain  Gain=4
  Gain2 : Gain  Gain=4
  Gain3 : Gain  Gain=1/2
  Reshape : Reshape  OutputDimensionality=Customize  OutputDimensions=[9,1]
  Sqrt : Sqrt
  Sum : Sum  Inputs=+-
  Sum1 : Sum  Inputs=++++
  Sum2 : Sum  Inputs=+-
  Sum3 : Sum  Inputs=+-
  Transpose1 : Math  Operator=transpose
  Vector Concatenate : Concatenate  NumInputs=4
  q-->DCM (CHECK) : Subsystem  Commented=on
  vector_norm : Subsystem
  q_B/N : Outport
  wires:
  A_B/N/1 -> Transpose1/1  "A_B/N"
  Transpose1/1 -> Reshape/1
  Divide3/1 -> q_B/N/1, q-->DCM (CHECK)/1(q_norm)  "q_norm"
  vector_norm/1(r_norm) -> Divide3/2
  Gain3/1 -> Vector Concatenate/4, Gain/1, Gain2/1, Gain1/1  "q4"
  Sqrt/1 -> Gain3/1
  Vector Concatenate/1 -> vector_norm/1(r), Divide3/1  "q"
  Gain2/1 -> Divide2/2
  Sum3/1 -> Divide2/1
  Gain1/1 -> Divide1/2
  Sum2/1 -> Divide1/1
  Gain/1 -> Divide/2
  Sum/1 -> Divide/1
  Constant/1 -> Sum1/1
  Sum1/1 -> Sqrt/1
  Divide2/1 -> Vector Concatenate/3  "q3"
  Divide1/1 -> Vector Concatenate/2  "q2"
  Divide/1 -> Vector Concatenate/1  "q1"
  Demux/9 -> Sum1/4  "A_33"
  Demux/8 -> Sum/2  "A_32"
  Demux/7 -> Sum2/1  "A_31"
  Demux/6 -> Sum/1  "A_23"
  Demux/5 -> Sum1/3  "A_22"
  Demux/4 -> Sum3/2  "A_21"
  Demux/3 -> Sum2/2  "A_13"
  Demux/2 -> Sum3/1  "A_12"
  Demux/1 -> Sum1/2  "A_11"
  Reshape/1 -> Demux/1

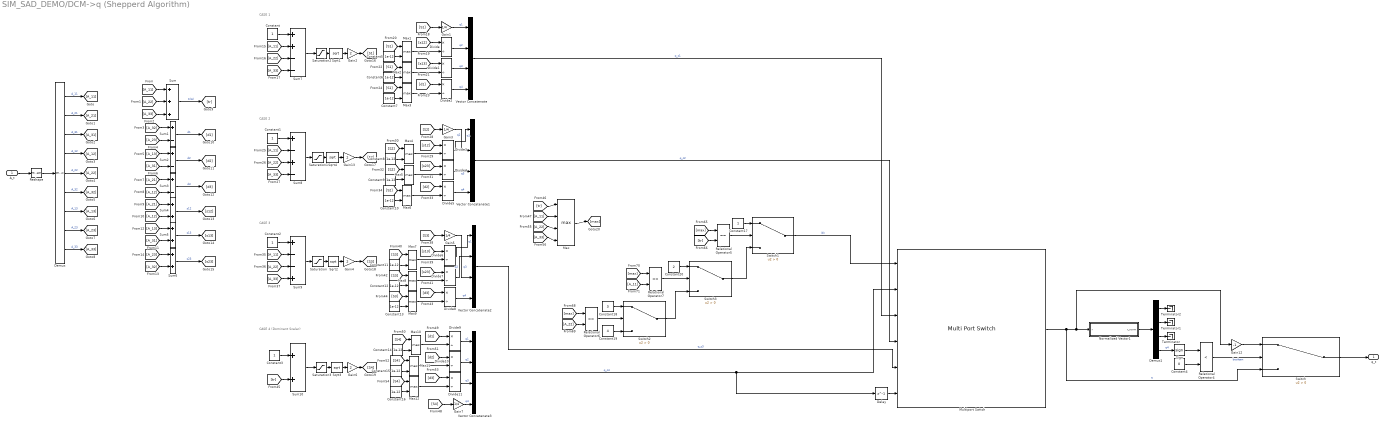
== system SIM_SAD_DEMO/DCM->q (Shepperd Algorithm) ==
  note: CASE 1
  note: CASE 2
  note: CASE 3
  note: CASE 4 (Dominant Scalar)
  A_t : Inport
  Constant{,1..3,17} (5 alike) : Constant
  Constant{5..16} (12 alike) : Constant  Value=1e-12
  Constant18 : Constant  Value=3
  Constant19 : Constant  Value=4
  Constant20 : Constant  Value=2
  Constant4 : Constant  Value=0
  Delay : Delay  DelayLength=1
  Demux : Demux  Outputs=9
  Demux1 : Demux
  Divide{,1..11} (12 alike) : Product  Inputs=*/
  Gain{1,3,5,7} (4 alike) : Gain  Gain=1/4
  Gain12 : Gain  Gain=-1
  Gain{2,4,6,13} (4 alike) : Gain  Gain=2
  Max : MinMax  Function=max  Inputs=4
  Max{1..12} (12 alike) : MinMax  Function=max  Inputs=2
  Multiport Switch : MultiPortSwitch  Inputs=4  DataPortForDefault=Additional data port  DiagnosticForDefault=Warning  SaturateOnIntegerOverflow=off
  Normalized Vector1 : Subsystem
  Relational Operator4 : RelationalOperator  Operator=<  OutDataTypeStr=boolean  RndMeth=Simplest  InputSameDT=off
  Relational Operator5 : RelationalOperator  Operator===  OutDataTypeStr=boolean  RndMeth=Simplest  InputSameDT=off
  Relational Operator6 : RelationalOperator  Operator===  OutDataTypeStr=boolean  RndMeth=Simplest  InputSameDT=off
  Relational Operator7 : RelationalOperator  Operator===  OutDataTypeStr=boolean  RndMeth=Simplest  InputSameDT=off
  Reshape : Reshape  OutputDimensionality=Customize  OutputDimensions=[9,1]
  Saturation{,1..3} (4 alike) : Saturate  UpperLimit=inf  LowerLimit=0
  Sign : Signum
  Sqrt{1..4} (4 alike) : Sqrt
  Sum : Sum  Inputs=+++
  Sum1 : Sum  Inputs=+-
  Sum{4..6,10} (4 alike) : Sum
  Sum2 : Sum  Inputs=+-
  Sum3 : Sum  Inputs=+-
  Sum7 : Sum  Inputs=++--
  Sum8 : Sum  Inputs=+-+-
  Sum9 : Sum  Inputs=+--+
  Switch{,1..3} (4 alike) : Switch  Criteria=u2 > Threshold  SaturateOnIntegerOverflow=off  InputSameDT=off
  Terminator : Terminator
  Terminator1 : Terminator
  Terminator2 : Terminator
  Vector Concatenate{,1..3} (4 alike) : Concatenate  NumInputs=4
  q_t : Outport
  wires:
  A_t/1 -> Reshape/1
  Reshape/1 -> Demux/1
  Demux/1 -> [A_11]  "A_11"
  Demux/2 -> [A_21]  "A_21"
  Demux/3 -> [A_31]  "A_31"
  Demux/4 -> [A_12]  "A_12"
  Demux/5 -> [A_22]  "A_22"
  Demux/6 -> [A_32]  "A_32"
  Demux/7 -> [A_13]  "A_13"
  Demux/8 -> [A_23]  "A_23"
  Demux/9 -> [A_33]  "A_33"
  Sum/1 -> [tr]  "tr(A)"
  [A_11] -> Sum/1
  [A_22] -> Sum/2
  [A_33] -> Sum/3
  [A_32] -> Sum1/1
  [A_23] -> Sum1/2
  Sum1/1 -> [d1]  "d1"
  Sum2/1 -> [d2]  "d2"
  [A_31] -> Sum2/2
  [A_13] -> Sum2/1
  [A_21] -> Sum3/1
  [A_12] -> Sum3/2
  Sum3/1 -> [d3]  "d3"
  Sum4/1 -> [s12]  "s12"
  [A_12] -> Sum4/2
  [A_21] -> Sum4/1
  [A_13] -> Sum5/1
  [A_31] -> Sum5/2
  Sum5/1 -> [s13]  "s13"
  Sum6/1 -> [s23]  "s23"
  [A_32] -> Sum6/2
  [A_23] -> Sum6/1
  [A_11] -> Sum7/2
  [A_22] -> Sum7/3
  [A_33] -> Sum7/4
  Constant/1 -> Sum7/1
  Sum7/1 -> Saturation2/1
  Gain2/1 -> [S1]
  [S1] -> Gain1/1
  Gain1/1 -> Vector Concatenate/1  "q1"
  [s12] -> Divide/1
  Divide/1 -> Vector Concatenate/2  "q2"
  Divide1/1 -> Vector Concatenate/3  "q3"
  [s13] -> Divide1/1
  [d1] -> Divide2/1
  Divide2/1 -> Vector Concatenate/4  "q4"
  Vector Concatenate/1 -> Multiport Switch/3  "q_c1"
  Vector Concatenate1/1 -> Multiport Switch/4  "q_c2"
  Divide5/1 -> Vector Concatenate1/4  "q4"
  [d2] -> Divide5/1
  [s23] -> Divide4/1
  Divide4/1 -> Vector Concatenate1/3  "q3"
  Divide3/1 -> Vector Concatenate1/1  "q1"
  [s12] -> Divide3/1
  Gain3/1 -> Vector Concatenate1/2  "q2"
  [S2] -> Gain3/1
  Gain13/1 -> [S2]
  Sum8/1 -> Saturation1/1
  Constant1/1 -> Sum8/1
  [A_33] -> Sum8/4
  [A_22] -> Sum8/3
  [A_11] -> Sum8/2
  [A_11] -> Sum9/2
  [A_22] -> Sum9/3
  [A_33] -> Sum9/4
  Constant2/1 -> Sum9/1
  Sum9/1 -> Saturation/1
  Sqrt2/1 -> Gain4/1
  Gain4/1 -> [S3]
  [S3] -> Gain5/1
  Gain5/1 -> Vector Concatenate2/3  "q3"
  [s13] -> Divide6/1
  Divide6/1 -> Vector Concatenate2/1  "q1"
  Divide7/1 -> Vector Concatenate2/2  "q2"
  Max8/1 -> Divide7/2
  [s23] -> Divide7/1
  [d3] -> Divide8/1
  Max9/1 -> Divide8/2
  Divide8/1 -> Vector Concatenate2/4  "q4"
  Vector Concatenate2/1 -> Multiport Switch/5  "q_c3"
  Vector Concatenate3/1 -> Multiport Switch/2, Delay/1  "q_c4"
  Divide11/1 -> Vector Concatenate3/3  "q3"
  [d3] -> Divide11/1
  [d2] -> Divide10/1
  Divide10/1 -> Vector Concatenate3/2  "q2"
  Divide9/1 -> Vector Concatenate3/1  "q1"
  [d1] -> Divide9/1
  Gain7/1 -> Vector Concatenate3/4  "q4"
  [S4] -> Gain7/1
  Gain6/1 -> [S4]
  Constant3/1 -> Sum10/1
  [tr] -> Sum10/2
  [tr] -> Max/1
  [A_11] -> Max/2
  [A_22] -> Max/3
  [A_33] -> Max/4
  Max/1 -> [max]
  Delay/1 -> Multiport Switch/6
  Multiport Switch/1 -> Switch/3, Gain12/1, Normalized Vector1/1(r)  "q"
  Normalized Vector1/1(r_norm) -> Demux1/1
  Demux1/4 -> Sign/1  "q4"
  Sign/1 -> Relational Operator4/1
  Demux1/3 -> Terminator/1
  Demux1/2 -> Terminator1/1
  Demux1/1 -> Terminator2/1
  Constant4/1 -> Relational Operator4/2
  Relational Operator4/1 -> Switch/2  "boolean"
  Gain12/1 -> Switch/1
  Switch/1 -> q_t/1
  Saturation/1 -> Sqrt2/1
  Saturation1/1 -> Sqrt4/1
  Sqrt4/1 -> Gain13/1
  Sqrt1/1 -> Gain2/1
  Saturation2/1 -> Sqrt1/1
  Saturation3/1 -> Sqrt3/1
  Sqrt3/1 -> Gain6/1
  Sum10/1 -> Saturation3/1
  [S1] -> Max1/1
  Constant5/1 -> Max1/2
  Max1/1 -> Divide/2
  Max2/1 -> Divide1/2
  Constant6/1 -> Max2/2
  [S1] -> Max2/1
  [S1] -> Max3/1
  Constant7/1 -> Max3/2
  Max3/1 -> Divide2/2
  [S2] -> Max4/1
  Constant8/1 -> Max4/2
  Max4/1 -> Divide3/2
  Max5/1 -> Divide4/2
  Constant9/1 -> Max5/2
  [S2] -> Max5/1
  [S2] -> Max6/1
  Constant10/1 -> Max6/2
  Max6/1 -> Divide5/2
  [S3] -> Max7/1
  Constant11/1 -> Max7/2
  Max7/1 -> Divide6/2
  Constant12/1 -> Max8/2
  [S3] -> Max8/1
  [S3] -> Max9/1
  Constant13/1 -> Max9/2
  Constant14/1 -> Max10/2
  [S4] -> Max10/1
  Max10/1 -> Divide9/2
  [S4] -> Max11/1
  Constant15/1 -> Max11/2
  Max11/1 -> Divide10/2
  Constant16/1 -> Max12/2
  [S4] -> Max12/1
  Max12/1 -> Divide11/2
  Relational Operator5/1 -> Switch1/2
  [tr] -> Relational Operator5/2
  [max] -> Relational Operator5/1
  Constant17/1 -> Switch1/1
  Switch3/1 -> Switch1/3
  Switch1/1 -> Multiport Switch/1  "idx"
  Constant18/1 -> Switch2/1
  Constant19/1 -> Switch2/3
  [max] -> Relational Operator6/1
  [A_22] -> Relational Operator6/2
  Relational Operator6/1 -> Switch2/2
  Relational Operator7/1 -> Switch3/2
  [A_11] -> Relational Operator7/2
  [max] -> Relational Operator7/1
  Constant20/1 -> Switch3/1
  Switch2/1 -> Switch3/3

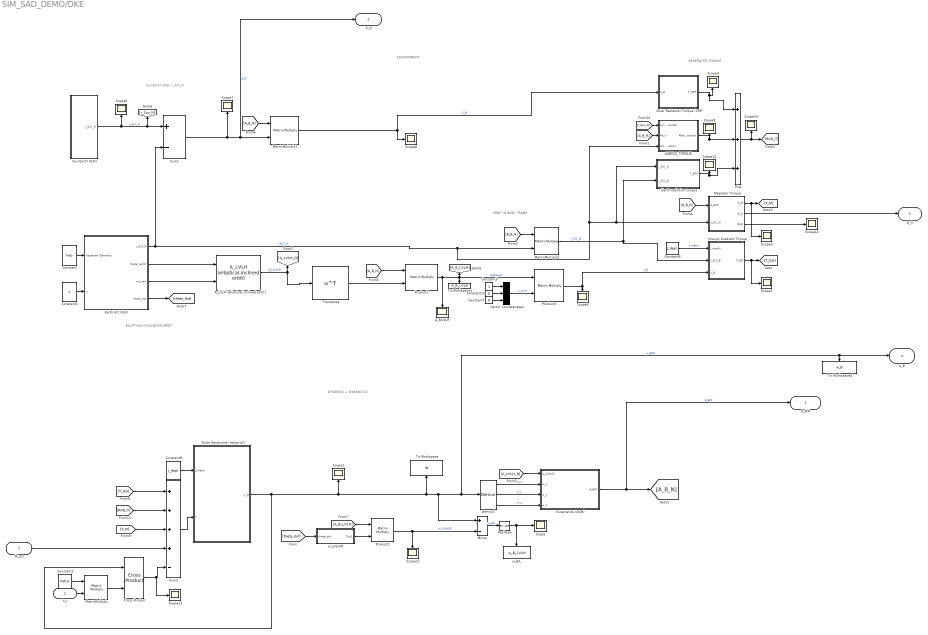
== system SIM_SAD_DEMO/DKE ==
  note: ORBIT IN BODY FRAME
  note: Sun-Earth Orbit r_S/C_N
  note: GENERATED TORQUE
  note: ELLIPTICAL INCLINATED ORBIT
  note: ENVIRONMENT
  note: DYNAMICS + KINEMATICS
  M_act : Inport
  h_r : Inport  Port=2
  ALBEDO_TORQUE : Subsystem
  A_B/LVLH : Scope
      settings: ActiveDisplayYMinimum=-0.55999388120508109  ActiveDisplayYMaximum=1.1733326534672313
  A_LVLH (elliptical,inclined orbit) : LIBRARY_SAD/A_LVLH (elliptical,inclined orbit)  SystemSampleTime=-1  VariantActivationTime=update diagram  EmptyChoice=off  PassThrough=off  PassThroughVariantControl=(default)  EmptyChoiceVariantControl=(default)  AllowFlexibleInterface=on  Latency=0  AutoFrameSizeCalculation=off
  Constant : Constant  Value=kep
  Constant1 : Constant  Value=n
  Constant10 : Constant  Value=0
  Constant2 : Constant  Value=RW.A
  Constant5 : Constant
  Constant7 : Constant  Value=0
  Constant8 : Constant  Value=J_depl
  Constant9 : Constant  Value=J_depl
  Cross Product : matrix_library/Cross Product
  Demux2 : Demux  Outputs=3
      settings: DisplayOption=none
  Earth radiation torque : Subsystem
  Earth-S/C Orbit : Subsystem
  Euler Equations (vectorial) : Subsystem
  Gravity Gradient Torque : Subsystem
  Kinematics (DCM) : Subsystem
  Magnetic Torque : Subsystem
  MatrixMultiply : Product  Multiplication=Matrix(*)
  MatrixMultiply1 : Product  Multiplication=Matrix(*)
  MatrixMultiply2 : Product  Multiplication=Matrix(*)
  Minus : Sum  Inputs=+-
  Plus : Sum  Inputs=+++
  Product1 : Product  Multiplication=Matrix(*)
  Product2 : Product  Multiplication=Matrix(*)
  Product3 : Product  Multiplication=Matrix(*)
  Reshape : Reshape  OutputDimensionality=Customize  OutputDimensions=[3,1]
  Scope{,1..14} (15 alike) : Scope
      Scope settings: ActiveDisplayYMinimum=-0.001958674555984172  ActiveDisplayYMaximum=0.00287841275217951
      Scope1 settings: ActiveDisplayYMinimum=-4.0939292859372782E-7  ActiveDisplayYMaximum=4.0997132442700667E-7  DataLoggingVariableName=ScopeData3
      Scope10 settings: ActiveDisplayYMinimum=-9.26278361948319E-8  ActiveDisplayYMaximum=4.4226864339294961E-8  DataLoggingVariableName=ScopeData27
      Scope11 settings: ActiveDisplayYMinimum=-1  ActiveDisplayYMaximum=1  DataLoggingVariableName=ScopeData21
      Scope12 settings: ActiveDisplayYMinimum=-2.1281934032262321E-8  ActiveDisplayYMaximum=2.2900279987034275E-8  DataLoggingVariableName=ScopeData9
      Scope13 settings: ActiveDisplayYMinimum=-0.0050393614618530272  ActiveDisplayYMaximum=0.0049475768856509193  DataLoggingVariableName=ScopeData108
      Scope14 settings: DataLoggingVariableName=ScopeData97
      Scope2 settings: ActiveDisplayYMinimum=-0.00013661573291137518  ActiveDisplayYMaximum=0.0012295415962023768  DataLoggingVariableName=ScopeData2
      Scope3 settings: ActiveDisplayYMinimum=-2.8956040019257018E-6  ActiveDisplayYMaximum=2.9066235698968462E-6  DataLoggingVariableName=ScopeData4
      Scope4 settings: ActiveDisplayYMinimum=-1  ActiveDisplayYMaximum=1  DataLoggingVariableName=ScopeData16
      Scope5 settings: ActiveDisplayYMinimum=-0.55998948749949928  ActiveDisplayYMaximum=1.1733321652777222  DataLoggingVariableName=ScopeData20
      Scope6 settings: ActiveDisplayYMinimum=-1  ActiveDisplayYMaximum=1  DataLoggingVariableName=ScopeData6
      Scope7 settings: ActiveDisplayYMinimum=-1  ActiveDisplayYMaximum=1  DataLoggingVariableName=ScopeData7
      Scope8 settings: ActiveDisplayYMinimum=-1  ActiveDisplayYMaximum=1  DataLoggingVariableName=ScopeData8
      Scope9 settings: ActiveDisplayYMinimum=-2.0339757656912845E-25  ActiveDisplayYMaximum=2.0339757656912845E-25  DataLoggingVariableName=ScopeData26
  Solar Radiation Torque (SRP) : Subsystem
  Sum1 : Sum  Inputs=+-
  Sum2 : Sum  Inputs=++++-
  Sun-Earth Orbit : Subsystem
  To Workspace : ToWorkspace  VariableName=w  SampleTime=-1
  To Workspace1 : ToWorkspace  VariableName=A_B_LVLH  SampleTime=-1
  To Workspace4 : ToWorkspace  VariableName=w_B  SampleTime=-1
  Transpose : Math  Operator=transpose
  Vector Concatenate2 : Concatenate  NumInputs=3
  w_B/L : ToWorkspace  VariableName=w_B_LVLH  SampleTime=-1
  w_LVLH/N : Subsystem
  A_B/N : Outport
  S_N : Outport  Port=2
  B_N : Outport  Port=3
  w_B : Outport  Port=4
  wires:
  Earth-S/C Orbit/2(theta_rad(t)) -> A_LVLH (elliptical,inclined orbit)/1
  Earth-S/C Orbit/3(incl_rad) -> A_LVLH (elliptical,inclined orbit)/2
  [A_B_N] -> MatrixMultiply2/1
  Sum2/1 -> Euler Equations (vectorial)/2(T)
  [A_B_N] -> ALBEDO_TORQUE/2(Ab_n)
  [A_B_N] -> MatrixMultiply1/1
  Demux2/3 -> Kinematics (DCM)/4(w_z)  "w_z"
  Kinematics (DCM)/1(A_B/N) -> A_B/N/1, [A_B_N]  "A_B/N"
  [T_M] -> Sum2/3
  Earth-S/C Orbit/4(theta_dot) -> [theta_dot]
  A_LVLH (elliptical,inclined orbit)/1 -> Transpose/1, [A_LVLH_N]  "A_LVLH/N"
  Demux2/1 -> Kinematics (DCM)/2(w_x)  "w_x"
  Earth radiation torque/1(T_ERP) -> Plus/3, Scope12/1
  [A_B_N] -> Product1/1
  Solar Radiation Torque (SRP)/1(T_SRP) -> Scope4/1, Plus/1
  MatrixMultiply1/1 -> Scope8/1, Solar Radiation Torque (SRP)/1(S_B)  "S_B"
  Constant7/1 -> Vector Concatenate2/3
  Constant10/1 -> Vector Concatenate2/2
  Constant9/1 -> Euler Equations (vectorial)/1(I_matrix)
  [A_LVLH_N] -> Kinematics (DCM)/1(A_LVLH/N)
  Constant8/1 -> Gravity Gradient Torque/1(I_matrix)  "I_matrix"
  Sum1/1 -> S_N/1, MatrixMultiply1/2, Scope7/1  "S_N"
  [RAD_T] -> Sum2/2
  Constant/1 -> Earth-S/C Orbit/1(Keplerian Elements)
  Constant1/1 -> Earth-S/C Orbit/2(n)
  [A_B_LVLH] -> Product2/1
  [r_Sun_N] -> ALBEDO_TORQUE/1(sun direction inertial)
  Product1/1 -> Product3/1, [A_B_LVLH], To Workspace1/1, A_B/LVLH/1  "A_B/LVLH"
  Transpose/1 -> Product1/2
  Product2/1 -> Minus/2, Scope11/1  "w_LVLH/B"
  Minus/1 -> Reshape/1  "w_B/L"
  w_LVLH/N/1(Out1) -> Product2/2
  Reshape/1 -> Scope/1, w_B/L/1
  ALBEDO_TORQUE/1(Albedo_torque) -> Scope9/1, Plus/2
  [T_GG] -> Sum2/1
  [A_B_N] -> Magnetic Torque/1(A_B/N)
  Earth-S/C Orbit/1(r_S/C_N) -> Sum1/2, ALBEDO_TORQUE/3(S/C direction), Magnetic Torque/2(r_S/C_N), Earth radiation torque/1(r_S/C_N), MatrixMultiply2/2  "r_S/C_N"
  Plus/1 -> [RAD_T], Scope10/1
  Euler Equations (vectorial)/1(w_B) -> Cross Product/1, To Workspace4/1, w_B/1, Demux2/1, Minus/1, To Workspace/1, Scope2/1  "w_B/N"
  Product3/1 -> Gravity Gradient Torque/3(c_B), Scope5/1  "c_B"
  Demux2/2 -> Kinematics (DCM)/3(w_y)  "w_y"
  Constant5/1 -> Vector Concatenate2/1
  Gravity Gradient Torque/1(T_GG) -> Scope1/1, [T_GG]
  MatrixMultiply2/1 -> Gravity Gradient Torque/2(r_S/C_B), Earth radiation torque/2(r_S/C_B)  "r_S/C_B"
  [theta_dot] -> w_LVLH/N/1(theta_dot)
  Magnetic Torque/1(T_M) -> Scope3/1, [T_M]
  Vector Concatenate2/1 -> Product3/2  "c_LVLH"
  Magnetic Torque/2(B_N) -> B_N/1
  Sun-Earth Orbit/1(r_Sun_N) -> Sum1/1, [r_Sun_N], Scope6/1  "r_Sun_N"
  Magnetic Torque/3(B_B) -> Scope14/1
  M_act/1 -> Sum2/4
  Constant2/1 -> MatrixMultiply/1
  h_r/1 -> MatrixMultiply/2
  MatrixMultiply/1 -> Cross Product/2
  Cross Product/1 -> Scope13/1, Sum2/5

== system SIM_SAD_DEMO/SENSORS ==
  w_B : Inport
  "B_N " : Inport  Port=2
  S_N : Inport  Port=3
  A_B/N : Inport  Port=4
  Divide : Product  Inputs=*/
  Divide1 : Product  Inputs=*/
  Divide2 : Product  Inputs=*/
  Gyroscope : Subsystem
  Magnetometer : Subsystem
  Sun Sensor : Subsystem
  To Workspace6 : ToWorkspace  VariableName=w_measured  SampleTime=-1
  vector_norm : LIBRARY_SAD/vector_norm  SystemSampleTime=-1  VariantActivationTime=update diagram  EmptyChoice=off  PassThrough=off  PassThroughVariantControl=(default)  EmptyChoiceVariantControl=(default)  AllowFlexibleInterface=on  Latency=0  AutoFrameSizeCalculation=off
  vector_norm1 : LIBRARY_SAD/vector_norm  SystemSampleTime=-1  VariantActivationTime=update diagram  EmptyChoice=off  PassThrough=off  PassThroughVariantControl=(default)  EmptyChoiceVariantControl=(default)  AllowFlexibleInterface=on  Latency=0  AutoFrameSizeCalculation=off
  vector_norm2 : LIBRARY_SAD/vector_norm  SystemSampleTime=-1  VariantActivationTime=update diagram  EmptyChoice=off  PassThrough=off  PassThroughVariantControl=(default)  EmptyChoiceVariantControl=(default)  AllowFlexibleInterface=on  Latency=0  AutoFrameSizeCalculation=off
  B_B_m : Outport
  S__N : Outport  Port=2
  B_N : Outport  Port=3
  s1_B : Outport  Port=4
  s2_B : Outport  Port=5
  w_B_m : Outport  Port=6
  wires:
  A_B/N/1 -> Sun Sensor/1(A_B/N), Magnetometer/2(A_B/N)
  S_N/1 -> S__N/1, vector_norm/1, Divide/1  "S_N"
  Divide/1 -> Sun Sensor/2(v1_N)  "S_N_hat"
  vector_norm/1 -> Divide/2
  "B_N "/1 -> Magnetometer/1(v2_N), B_N/1
  vector_norm1/1 -> Divide1/2
  Divide1/1 -> s2_B/1
  vector_norm2/1 -> Divide2/2
  Divide2/1 -> s1_B/1
  Gyroscope/1(w_m) -> w_B_m/1, To Workspace6/1
  w_B/1 -> Gyroscope/1(w_B (rad/s))
  Magnetometer/1(s2_B) -> B_B_m/1, Divide1/1, vector_norm1/1
  Sun Sensor/1(s1_B) -> Divide2/1, vector_norm2/1

== system SIM_SAD_DEMO/STATE-SPACE VECTOR ==
  w_est : Inport
  A_B/T_e : Inport  Port=2
  Demux : Demux  Outputs=9
  Gain : Gain  Gain=0.5
  Gain1 : Gain  Gain=0.5
  Gain2 : Gain  Gain=0.5
  Reshape : Reshape  OutputDimensionality=Customize  OutputDimensions=[9,1]
  Sum : Sum  Inputs=+-
  Sum1 : Sum  Inputs=+-
  Sum2 : Sum  Inputs=+-
  Terminator : Terminator
  Terminator1 : Terminator
  Terminator2 : Terminator
  To Workspace : ToWorkspace  VariableName=x  SampleTime=-1
  Vector Concatenate : Concatenate  NumInputs=3
  Vector Concatenate1 : Concatenate
  x : Outport
  wires:
  A_B/T_e/1 -> Reshape/1
  Reshape/1 -> Demux/1
  Demux/1 -> Terminator1/1  "A_11"
  Demux/2 -> Sum2/2  "A_21"
  Demux/3 -> Sum1/1  "A_31"
  Demux/4 -> Sum2/1  "A_12"
  Demux/5 -> Terminator/1  "A_22"
  Demux/6 -> Sum/2  "A_32"
  Demux/7 -> Sum1/2  "A_13"
  Demux/8 -> Sum/1  "A_23"
  Demux/9 -> Terminator2/1  "A_33"
  Sum/1 -> Gain/1
  Sum1/1 -> Gain1/1
  Sum2/1 -> Gain2/1
  Gain/1 -> Vector Concatenate/1  "x1"
  Gain1/1 -> Vector Concatenate/2  "x2"
  Gain2/1 -> Vector Concatenate/3  "x3"
  Vector Concatenate/1 -> Vector Concatenate1/2
  w_est/1 -> Vector Concatenate1/1  "x1,x2,x3"
  Vector Concatenate1/1 -> To Workspace/1, x/1  "x"
